simulink model "hw2_hvac"  (R2014a)
settings: Solver=ode45  StartTime=0.0  StopTime=inf  RelTol=1e-3
settings Model: Creator=feisele  LastModifiedBy=feisele

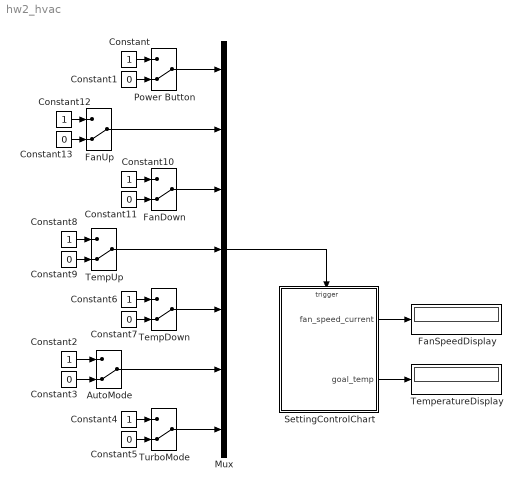
== system hw2_hvac ==
  AutoMode : ManualSwitch  CurrentSetting=0
  Constant{,2,4,6,8,10,12} (7 alike) : Constant
  Constant{1,3,5,7,9,11,13} (7 alike) : Constant  Value=0
  FanDown : ManualSwitch  CurrentSetting=0
  FanSpeedDisplay : Display
  FanUp : ManualSwitch  CurrentSetting=0
  Mux : Mux  Inputs=7
  Power Button : ManualSwitch  CurrentSetting=0
  SettingControlChart : Stateflow chart  TreatAsAtomicUnit=on
  TempDown : ManualSwitch  CurrentSetting=0
  TempUp : ManualSwitch  CurrentSetting=0
  TemperatureDisplay : Display
  TurboMode : ManualSwitch  CurrentSetting=0
  wires:
  Power Button/1 -> Mux/1
  Constant/1 -> Power Button/1
  SettingControlChart/1(fan_speed_current) -> FanSpeedDisplay/1
  SettingControlChart/2(goal_temp) -> TemperatureDisplay/1
  FanUp/1 -> Mux/2
  Mux/1 -> SettingControlChart/Trigger
  FanDown/1 -> Mux/3
  TempUp/1 -> Mux/4
  TempDown/1 -> Mux/5
  Constant2/1 -> AutoMode/1
  Constant3/1 -> AutoMode/2
  Constant4/1 -> TurboMode/1
  Constant5/1 -> TurboMode/2
  AutoMode/1 -> Mux/6
  TurboMode/1 -> Mux/7
  Constant6/1 -> TempDown/1
  Constant7/1 -> TempDown/2
  Constant8/1 -> TempUp/1
  Constant9/1 -> TempUp/2
  Constant10/1 -> FanDown/1
  Constant11/1 -> FanDown/2
  Constant12/1 -> FanUp/1
  Constant13/1 -> FanUp/2
  Constant1/1 -> Power Button/2

== stateflow chart hw2_hvac/SettingControlChart ==
  settings: executeAtInitialization=1
  state Power_off
  state Power_on
    state Temperature_setting [parallel]
      settings: executionOrder=1
      state Temp
      (junction 66) -> (junction 67) [order 2] : temp_up
          | [goal_temp < MAXT]
          | { manual_temp = manual_temp + 1; }
      Temp -> (junction 66) : [not(in(Mode.Computed.Auto))]
      (junction 66) -> (junction 67) [order 1] : temp_down
          | [MINT < goal_temp]
          | { manual_temp = manual_temp - 1; }
      (default) -> Temp
      (junction 67) -> Temp : { goal_temp = manual_temp; }
    state Mode [parallel]
      settings: executionOrder=2
      (history)
      state Manual
      state Computed
        (history)
        state Auto
        state Turbo
        (junction 70) -> Auto : { fan_speed_current = AUTO_FAN; }
        (default) -> (junction 70)
      (junction 55) -> Manual : { fan_speed_current = manual_fan;
          | goal_temp = manual_temp; }
      Computed -> (junction 55) [order 2] : fan_down
      Computed -> (junction 55) [order 1] : fan_up
      (default) -> Computed
      Mode -> (junction 70) [order 2] : auto_on
          | { goal_temp = manual_temp; }
      Mode -> Turbo [order 1] : turbo_on
          | { goal_temp = MAXT;
          | fan_speed_current = MAXF; }
    state Fan_setting [parallel]
      settings: executionOrder=3
      state Fan
      (junction 58) -> (junction 62) [order 1] : fan_up
          | [ fan_speed_current < MAXF]
          | { manual_fan = manual_fan + 1; }
      (junction 58) -> (junction 62) [order 2] : fan_down
          | [MINF < fan_speed_current]
          | { manual_fan = manual_fan - 1; }
      Fan -> (junction 58) : [ in(Mode.Manual)]
      (default) -> Fan
      (junction 62) -> Fan : { fan_speed_current = manual_fan; }
  (default) -> Power_off : {manual_fan = AUTO_FAN;
      |  manual_temp = MAXT;
      | fan_speed_current  = manual_fan;
      | goal_temp = manual_temp; }
  Power_on -> Power_off : power_press
  Power_off -> Power_on : power_press
  data: MAXF constant int8 =10; MINF constant int8 =0; MINT constant int8 =0; MAXT constant int8 =30; fan_speed_current output int8; goal_temp output int8; manual_fan local int8 =5; manual_temp local int8 =10; AUTO_FAN constant int8 =7
  events: power_press input EITHER_EDGE_EVENT; fan_up input EITHER_EDGE_EVENT; fan_down input EITHER_EDGE_EVENT; temp_up input EITHER_EDGE_EVENT; temp_down input EITHER_EDGE_EVENT; auto_on input EITHER_EDGE_EVENT; turbo_on input EITHER_EDGE_EVENT
